simulink model "ysw11_9"  (R2014a)
settings: Solver=ode45  StartTime=0.0  StopTime=10.0  RelTol=1e-3
libraries: commanapbnd3 x1
settings Model: Creator=ii  LastModifiedBy=ii
settings SolverCC: ZeroCrossAlgorithm=Adaptive
settings DebuggingCC: UnderspecifiedInitializationDetection=Classic

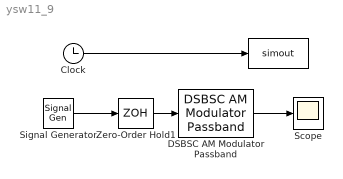
== system ysw11_9 ==
  "  " : ToWorkspace  VariableName=simout  SampleTime=-1
  Clock : Clock
  DSBSC AM Modulator Passband : commanapbnd3/DSBSC AM Modulator Passband  Fc=300  Ph=pi/3
  Scope : Scope
  Signal Generator : SignalGenerator  Frequency=700  Units=rad/sec
  Zero-Order Hold1 : ZeroOrderHold
  wires:
  Clock/1 -> "  "/1
  Signal Generator/1 -> Zero-Order Hold1/1
  Zero-Order Hold1/1 -> DSBSC AM Modulator Passband/1
  DSBSC AM Modulator Passband/1 -> Scope/1
